simulink model "lab1"  (R2016b)
settings: Solver=VariableStepAuto  StartTime=0.0  StopTime=50  RelTol=1e-3
settings Model: Creator=guilherme.mercurio  LastModifiedBy=guilherme.mercurio

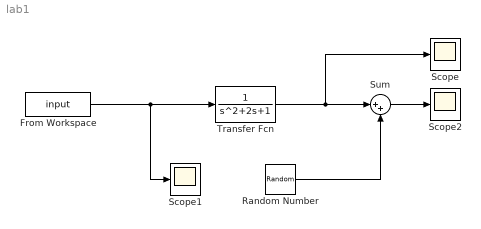
== system lab1 ==
  From Workspace : FromWorkspace  VariableName=input
  Random Number : RandomNumber  Variance=0.01  SampleTime=0.1
  Scope : Scope
  Scope1 : Scope
  Scope2 : Scope
  Sum : Sum  Inputs=|++
  Transfer Fcn : TransferFcn
  wires:
  Random Number/1 -> Sum/2
  Transfer Fcn/1 -> Scope/1, Sum/1
  Sum/1 -> Scope2/1
  From Workspace/1 -> Scope1/1, Transfer Fcn/1
